simulink model "Ex06"  (R2021b)
settings: Solver=VariableStepAuto  StartTime=0.0  StopTime=10  MaxStep=1e-3  RelTol=1e-3
settings Model: Creator=carlo  LastModifiedBy=carlo
settings SolverCC: AlgebraicLoopSolver=TrustRegion
settings DebuggingCC: SFMachineParentedDataDiag=warning

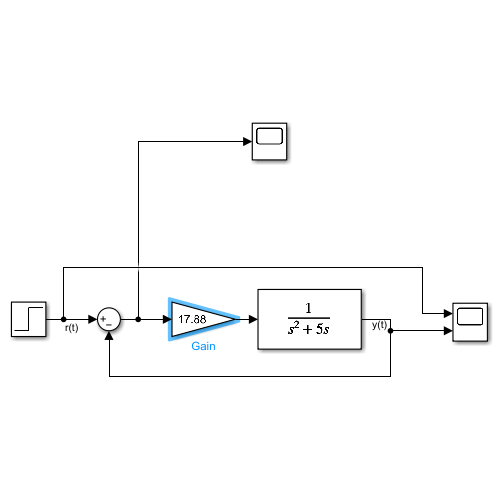
[thumbnail: Simulink's stored preview of the top-level diagram]
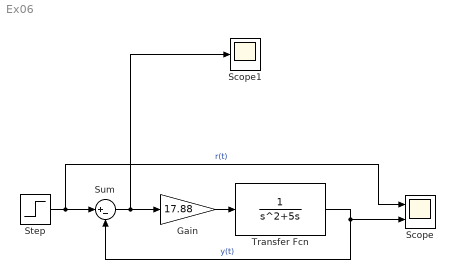
== system Ex06 ==
  Gain : Gain  Gain=17.88
  Scope : Scope  NumInputPorts=2
  Scope1 : Scope
  Step : Step  SampleTime=0
  Sum : Sum  Inputs=|+-
  Transfer Fcn : TransferFcn  Denominator=[1 5 0]
  wires:
  Gain/1 -> Transfer Fcn/1
  Sum/1 -> Scope1/1, Gain/1
  Transfer Fcn/1 -> Scope/2, Sum/2  "y(t)"
  Step/1 -> Scope/1, Sum/1  "r(t)"
